simulink subsystem "Sonares"  (R2023b)
settings: Solver=VariableStepAuto  StartTime=0.0  StopTime=10.0  RelTol=1e-3
libraries: arduinolib x2
settings Model: Creator=Andrés  LastModifiedBy=Andrés

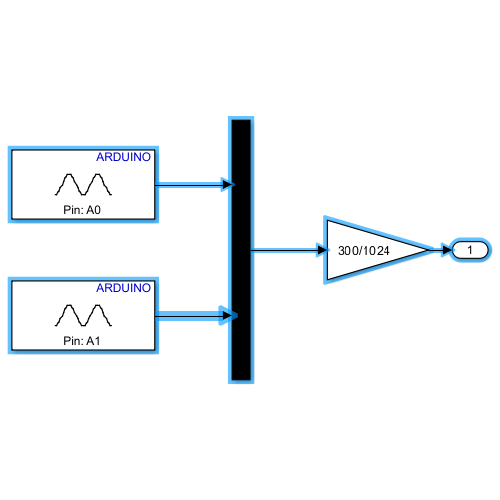
[thumbnail: Simulink's stored preview of the top-level diagram]
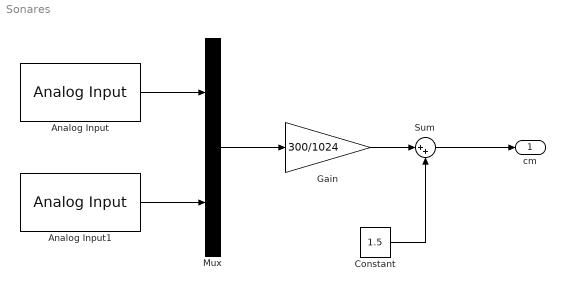
== system Sonares ==
  Analog Input : arduinolib/Analog Input  pinNumber=1  ReadResultsOnly=off  ConversionTriggerSource=Software  ExternalTriggerType=uint32( 0 )  OutputDataType=uint16  EnableConversionCompleteNotify=off  EnableOuputStatus=off  SampleTime=-1  blockPlatform=arduino
  Analog Input1 : arduinolib/Analog Input  pinNumber=2  ReadResultsOnly=off  ConversionTriggerSource=Software  ExternalTriggerType=uint32( 0 )  OutputDataType=uint16  EnableConversionCompleteNotify=off  EnableOuputStatus=off  SampleTime=-1  blockPlatform=arduino
  Constant : Constant  Value=1.5
  Gain : Gain  Gain=300/1024
  Mux : Mux  Inputs=2
  Sum : Sum  Inputs=|++
  cm : Outport
  wires:
  Analog Input/1 -> Mux/1
  Mux/1 -> Gain/1
  Analog Input1/1 -> Mux/2
  Gain/1 -> Sum/1
  Sum/1 -> cm/1
  Constant/1 -> Sum/2
